simulink model "ES008A_PwrSply"  (R2013b)
settings: Solver=FixedStepDiscrete  SolverMode=SingleTasking  StartTime=0.0  StopTime=1  FixedStep=0.002  RelTol=1e-3
values from neighbouring files (symbols this model uses):
  DiagcReg0Err = DataDict.NTC    [ES008A_PwrSply_DataDict.m]
  DiagcReg1Err = DataDict.NTC    [ES008A_PwrSply_DataDict.m]
  PWRSPLYDIAGREG0READVAL_CNT_U16 = DataDict.Constant    [ES008A_PwrSply_DataDict.m]
  PWRSPLYDIAGREG1READVAL_CNT_U16 = DataDict.Constant    [ES008A_PwrSply_DataDict.m]
  PwrSplyNtc0x07BFailStep = DataDict.Calibration    [ES008A_PwrSply_DataDict.m]
  PwrSplyNtc0x07BPassStep = DataDict.Calibration    [ES008A_PwrSply_DataDict.m]
  PwrSplyNtc0x07CFailStep = DataDict.Calibration    [ES008A_PwrSply_DataDict.m]
  PwrSplyNtc0x07CPassStep = DataDict.Calibration    [ES008A_PwrSply_DataDict.m]
  PwrSplyNtc0x07DFailStep = DataDict.Calibration    [ES008A_PwrSply_DataDict.m]
  PwrSplyNtc0x07DPassStep = DataDict.Calibration    [ES008A_PwrSply_DataDict.m]
  PWRSPLYOUTPENAWRVAL_CNT_U16 = DataDict.Constant    [ES008A_PwrSply_DataDict.m]
  PWRSPLYVRFYRESREG0READVAL_CNT_U16 = DataDict.Constant    [ES008A_PwrSply_DataDict.m]
  PWRSPLYVRFYRESREG1READVAL_CNT_U16 = DataDict.Constant    [ES008A_PwrSply_DataDict.m]
  SerlErr = DataDict.NTC    [ES008A_PwrSply_DataDict.m]
  SpiConf_SpiChannel_PwrSplyCh1 = DataDict.Constant    [ES008A_PwrSply_DataDict.m]
  SpiConf_SpiChannel_PwrSplyCh2 = DataDict.Constant    [ES008A_PwrSply_DataDict.m]
  SpiConf_SpiChannel_PwrSplyCh3 = DataDict.Constant    [ES008A_PwrSply_DataDict.m]
  SpiConf_SpiChannel_PwrSplyCh4 = DataDict.Constant    [ES008A_PwrSply_DataDict.m]
  SpiConf_SpiChannel_PwrSplyCh5 = DataDict.Constant    [ES008A_PwrSply_DataDict.m]
  SpiConf_SpiSequence_PwrSplySeq1 = DataDict.Constant    [ES008A_PwrSply_DataDict.m]
  SpiConf_SpiSequence_PwrSplySeq2 = DataDict.Constant    [ES008A_PwrSply_DataDict.m]
  SpiConf_SpiSequence_PwrSplySeq3 = DataDict.Constant    [ES008A_PwrSply_DataDict.m]
  SpiConf_SpiSequence_PwrSplySeq4 = DataDict.Constant    [ES008A_PwrSply_DataDict.m]
  SpiConf_SpiSequence_PwrSplySeq5 = DataDict.Constant    [ES008A_PwrSply_DataDict.m]
  StrtUpSelfTestReg0Err = DataDict.NTC    [ES008A_PwrSply_DataDict.m]
  StrtUpSelfTestReg1Err = DataDict.NTC    [ES008A_PwrSply_DataDict.m]
undefined symbols (not defined in the file or in its folder): sigbuilder_block, SysSt1
libraries: simulink x11
(part 3 of 4)

== system ES008A_PwrSply/PwrSply/PwrSplyPer1/SysSt = Warm Init OR Enable/PwrSplyReadWrOrderFlg2 = 0 (Write Cmd to get Diag Status) /Read Message 1/Call_Spi_AsyncTransmit ==
  Sequence : Inport
  CopyRight1 : Subsystem  Description=|  mask(Copyright Information){none=on}
      | Copyright info block.                                               
      |                                                                     
      | Place copyright information at the top of every subsystem in design.
      mask prompts: none "No parameters"
      mask help: Place copyright information at the top of every subsystem in design.
      mask Display:
      | NxtrConf = 'Nexteer Confidential';
      | 
      | sys = bdroot; %handle for the current model ("system")
      | first = get_param(sys,'Created');
      | first = first(end-3:end);  %year is last four digits
      | 
      | last = get_param(sys,'LastModifiedDate');
      | if isempty(last)
      |     last = datestr(now,'yyyy');
      | else
      |     last = last(end-3:end);
      | end
      | 
      | if strcmp(first,last)
      |     fprintf('%s -- Copyright %s Nexteer',NxtrConf,first)
      | else
      |     fprintf('%s -- %s%s- %s Nexteer',NxtrConf,char(169),first,last)
      | end
  Terminator : Terminator
  wires:
  Sequence/1 -> Terminator/1

== system ES008A_PwrSply/PwrSply/PwrSplyPer1/SysSt = Warm Init OR Enable/PwrSplyReadWrOrderFlg2 = 0 (Write Cmd to get Diag Status) /Read Message 1/CopyRight1 ==

== system ES008A_PwrSply/PwrSply/PwrSplyPer1/SysSt = Warm Init OR Enable/PwrSplyReadWrOrderFlg2 = 0 (Write Cmd to get Diag Status) /Read Message 1/Spi_WriteIB ==
  Channel : Inport
  DataBufferPtr : Inport  Port=2
  CopyRight1 : Subsystem  Description=|  mask(Copyright Information){none=on}
      | Copyright info block.                                               
      |                                                                     
      | Place copyright information at the top of every subsystem in design.
      mask prompts: none "No parameters"
      mask help: Place copyright information at the top of every subsystem in design.
      mask Display:
      | NxtrConf = 'Nexteer Confidential';
      | 
      | sys = bdroot; %handle for the current model ("system")
      | first = get_param(sys,'Created');
      | first = first(end-3:end);  %year is last four digits
      | 
      | last = get_param(sys,'LastModifiedDate');
      | if isempty(last)
      |     last = datestr(now,'yyyy');
      | else
      |     last = last(end-3:end);
      | end
      | 
      | if strcmp(first,last)
      |     fprintf('%s -- Copyright %s Nexteer',NxtrConf,first)
      | else
      |     fprintf('%s -- %s%s- %s Nexteer',NxtrConf,char(169),first,last)
      | end
  Terminator : Terminator
  Terminator1 : Terminator
  wires:
  DataBufferPtr/1 -> Terminator1/1
  Channel/1 -> Terminator/1

== system ES008A_PwrSply/PwrSply/PwrSplyPer1/SysSt = Warm Init OR Enable/PwrSplyReadWrOrderFlg2 = 0 (Write Cmd to get Diag Status) /Read Message 2/Call_Spi_AsyncTransmit ==
  Sequence : Inport
  CopyRight1 : Subsystem  Description=|  mask(Copyright Information){none=on}
      | Copyright info block.                                               
      |                                                                     
      | Place copyright information at the top of every subsystem in design.
      mask prompts: none "No parameters"
      mask help: Place copyright information at the top of every subsystem in design.
      mask Display:
      | NxtrConf = 'Nexteer Confidential';
      | 
      | sys = bdroot; %handle for the current model ("system")
      | first = get_param(sys,'Created');
      | first = first(end-3:end);  %year is last four digits
      | 
      | last = get_param(sys,'LastModifiedDate');
      | if isempty(last)
      |     last = datestr(now,'yyyy');
      | else
      |     last = last(end-3:end);
      | end
      | 
      | if strcmp(first,last)
      |     fprintf('%s -- Copyright %s Nexteer',NxtrConf,first)
      | else
      |     fprintf('%s -- %s%s- %s Nexteer',NxtrConf,char(169),first,last)
      | end
  Terminator : Terminator
  wires:
  Sequence/1 -> Terminator/1

== system ES008A_PwrSply/PwrSply/PwrSplyPer1/SysSt = Warm Init OR Enable/PwrSplyReadWrOrderFlg2 = 0 (Write Cmd to get Diag Status) /Read Message 2/CopyRight1 ==

== system ES008A_PwrSply/PwrSply/PwrSplyPer1/SysSt = Warm Init OR Enable/PwrSplyReadWrOrderFlg2 = 0 (Write Cmd to get Diag Status) /Read Message 2/Spi_WriteIB ==
  Channel : Inport
  DataBufferPtr : Inport  Port=2
  CopyRight1 : Subsystem  Description=|  mask(Copyright Information){none=on}
      | Copyright info block.                                               
      |                                                                     
      | Place copyright information at the top of every subsystem in design.
      mask prompts: none "No parameters"
      mask help: Place copyright information at the top of every subsystem in design.
      mask Display:
      | NxtrConf = 'Nexteer Confidential';
      | 
      | sys = bdroot; %handle for the current model ("system")
      | first = get_param(sys,'Created');
      | first = first(end-3:end);  %year is last four digits
      | 
      | last = get_param(sys,'LastModifiedDate');
      | if isempty(last)
      |     last = datestr(now,'yyyy');
      | else
      |     last = last(end-3:end);
      | end
      | 
      | if strcmp(first,last)
      |     fprintf('%s -- Copyright %s Nexteer',NxtrConf,first)
      | else
      |     fprintf('%s -- %s%s- %s Nexteer',NxtrConf,char(169),first,last)
      | end
  Terminator : Terminator
  Terminator1 : Terminator
  wires:
  Channel/1 -> Terminator/1
  DataBufferPtr/1 -> Terminator1/1

== system ES008A_PwrSply/PwrSply/PwrSplyPer1/SysSt = Warm Init OR Enable/PwrSplyReadWrOrderFlg2 = 1 (Read Buffer)/Channel 4/CH 4 // Verify Result Reg 0 - NTCNR_0X07E (V5A, V5CAN, 3V3, BUCK) ==
  note: Channel 4 --> for Verify_Result_0 Register
      | Channel 5 --> for Verify_Result_1 Register
  NtcStsInfo : Inport
  Action Port : ActionPort  ActionType=then
  Bitwise Operator1 : simulink/Logic and Bit Operations/Bitwise Operator  logicop=NOT  UseBitMask=off  BitMask=bin2dec('11011001')  BitMaskRealWorld=Stored Integer
  CopyRight1 : Subsystem  Description=|  mask(Copyright Information){none=on}
      | Copyright info block.                                               
      |                                                                     
      | Place copyright information at the top of every subsystem in design.
      mask prompts: none "No parameters"
      mask help: Place copyright information at the top of every subsystem in design.
      mask Display:
      | NxtrConf = 'Nexteer Confidential';
      | 
      | sys = bdroot; %handle for the current model ("system")
      | first = get_param(sys,'Created');
      | first = first(end-3:end);  %year is last four digits
      | 
      | last = get_param(sys,'LastModifiedDate');
      | if isempty(last)
      |     last = datestr(now,'yyyy');
      | else
      |     last = last(end-3:end);
      | end
      | 
      | if strcmp(first,last)
      |     fprintf('%s -- Copyright %s Nexteer',NxtrConf,first)
      | else
      |     fprintf('%s -- %s%s- %s Nexteer',NxtrConf,char(169),first,last)
      | end
  Ground : Ground
  NtcNr : Constant  Value=StrtUpSelfTestReg0Err
  NtcSts : Constant  OutDataTypeStr=uint8
  SetNtcSts : Subsystem  RequirementInfo={'linktype_rmi_doors' '0000cf50 (/ESG Group/FDD Module Requirements/EA4 Specific/ES008A_PwrSply)' '#ES008A_128' 'true' 'REQ: ES008A_128' '' ; 'linktype_rmi_doors' '0000cf50 (/ESG Group/FDD Module Requirements/EA4 Specific/ES008A_PwrSply)' '#ES008A_129' 'true' 'REQ: ES008A_129' '' ; 'linktype_rmi_doors' '0000cf50 (/ESG Group/FDD Module Requirements/EA4 Specific/ES008A_PwrSply)' '#ES008A_135' 'true' 'REQ: ES008A_135' '' ; 'linktype_rmi_doors' '0000cf50 (/ESG Group/FDD Module Requirements/EA4 Specific/ES008A_PwrSply)' '#ES008A_134' 'true' 'REQ: ES008A_134' '' ; 'linktype_rmi_doors' '0000cf50 (/ESG Group/FDD Module Requirements/EA4 Specific/ES008A_PwrSply)' '#ES008A_133' 'true' 'REQ: ES008A_133' '' ; 'linktype_rmi_doors' '0000cf50 (/ESG Group/FDD Module Requirements/EA4 Specific/ES008A_PwrSply)' '#ES008A_132' 'true' 'REQ: ES008A_132' '' ; 'linktype_rmi_doors' '0000cf50 (/ESG Group/FDD Module Requirements/EA4 Specific/ES008A_PwrSply)' '#ES008A_131' 'true' 'REQ: ES008A_131' '' ; 'linktype_rmi_doors' '0000cf50 (/ESG Group/FDD Module Requirements/EA4 Specific/ES008A_PwrSply)' '#ES008A_130' 'true' 'REQ: ES008A_130' '' } %GIDa_275bfab4_ec12_4082_a419_c11eb7b6dec0
  wires:
  NtcStsInfo/1 -> Bitwise Operator1/1
  Ground/1 -> SetNtcSts/4(DebStep)
  NtcSts/1 -> SetNtcSts/3(NtcSts)
  Bitwise Operator1/1 -> SetNtcSts/2(NtcStInfo)
  NtcNr/1 -> SetNtcSts/1(NtcNr)

== system ES008A_PwrSply/PwrSply/PwrSplyPer1/SysSt = Warm Init OR Enable/PwrSplyReadWrOrderFlg2 = 1 (Read Buffer)/Channel 4/CopyRight1 ==

== system ES008A_PwrSply/PwrSply/PwrSplyPer1/SysSt = Warm Init OR Enable/PwrSplyReadWrOrderFlg2 = 1 (Read Buffer)/Channel 4/No Startup Test Error 0 ==
  Action Port : ActionPort  ActionType=else
  CopyRight1 : Subsystem  Description=|  mask(Copyright Information){none=on}
      | Copyright info block.                                               
      |                                                                     
      | Place copyright information at the top of every subsystem in design.
      mask prompts: none "No parameters"
      mask help: Place copyright information at the top of every subsystem in design.
      mask Display:
      | NxtrConf = 'Nexteer Confidential';
      | 
      | sys = bdroot; %handle for the current model ("system")
      | first = get_param(sys,'Created');
      | first = first(end-3:end);  %year is last four digits
      | 
      | last = get_param(sys,'LastModifiedDate');
      | if isempty(last)
      |     last = datestr(now,'yyyy');
      | else
      |     last = last(end-3:end);
      | end
      | 
      | if strcmp(first,last)
      |     fprintf('%s -- Copyright %s Nexteer',NxtrConf,first)
      | else
      |     fprintf('%s -- %s%s- %s Nexteer',NxtrConf,char(169),first,last)
      | end
  Ground : Ground
  NtcNr : Constant  Value=StrtUpSelfTestReg0Err
  NtcSts : Constant  Value=0  OutDataTypeStr=uint8
  NtcStsInfo : Constant  Value=0  OutDataTypeStr=uint8
  SetNtcSts : Subsystem  RequirementInfo={'linktype_rmi_doors' '0000cf50 (/ESG Group/FDD Module Requirements/EA4 Specific/ES008A_PwrSply)' '#ES008A_124' 'true' 'REQ: ES008A_124' '' } %GIDa_e0576653_0d47_4805_9c34_52b8011502e8
  wires:
  NtcStsInfo/1 -> SetNtcSts/2(NtcStInfo)
  NtcNr/1 -> SetNtcSts/1(NtcNr)
  Ground/1 -> SetNtcSts/4(DebStep)
  NtcSts/1 -> SetNtcSts/3(NtcSts)

== system ES008A_PwrSply/PwrSply/PwrSplyPer1/SysSt = Warm Init OR Enable/PwrSplyReadWrOrderFlg2 = 1 (Read Buffer)/Channel 4/Spi_ReadIB ==
  note: Read Buffer - Simulation Purpose Only
      |
      |
      |
      |               XXXX XXXX 1111 1111
  note: 001011111111110
  Channel : Inport
  Constant3 : Constant  Value=255  OutDataTypeStr=uint16
  CopyRight1 : Subsystem  Description=|  mask(Copyright Information){none=on}
      | Copyright info block.                                               
      |                                                                     
      | Place copyright information at the top of every subsystem in design.
      mask prompts: none "No parameters"
      mask help: Place copyright information at the top of every subsystem in design.
      mask Display:
      | NxtrConf = 'Nexteer Confidential';
      | 
      | sys = bdroot; %handle for the current model ("system")
      | first = get_param(sys,'Created');
      | first = first(end-3:end);  %year is last four digits
      | 
      | last = get_param(sys,'LastModifiedDate');
      | if isempty(last)
      |     last = datestr(now,'yyyy');
      | else
      |     last = last(end-3:end);
      | end
      | 
      | if strcmp(first,last)
      |     fprintf('%s -- Copyright %s Nexteer',NxtrConf,first)
      | else
      |     fprintf('%s -- %s%s- %s Nexteer',NxtrConf,char(169),first,last)
      | end
  Terminator : Terminator
  Rx : Outport
  wires:
  Channel/1 -> Terminator/1
  Constant3/1 -> Rx/1

== system ES008A_PwrSply/PwrSply/PwrSplyPer1/SysSt = Warm Init OR Enable/PwrSplyReadWrOrderFlg2 = 1 (Read Buffer)/Channel 5/CH 5 // Verify Result Reg 1 - NTCNR_0X07F (VREG, V5P, V5B) ==
  note: Channel 4 --> for Verify_Result_0 Register
      | Channel 5 --> for Verify_Result_1 Register
  NtcStsInfo : Inport
  Action Port : ActionPort  ActionType=then
  Bitwise Operator1 : simulink/Logic and Bit Operations/Bitwise Operator  logicop=NOT  UseBitMask=off  BitMask=bin2dec('11011001')  BitMaskRealWorld=Stored Integer
  CopyRight1 : Subsystem  Description=|  mask(Copyright Information){none=on}
      | Copyright info block.                                               
      |                                                                     
      | Place copyright information at the top of every subsystem in design.
      mask prompts: none "No parameters"
      mask help: Place copyright information at the top of every subsystem in design.
      mask Display:
      | NxtrConf = 'Nexteer Confidential';
      | 
      | sys = bdroot; %handle for the current model ("system")
      | first = get_param(sys,'Created');
      | first = first(end-3:end);  %year is last four digits
      | 
      | last = get_param(sys,'LastModifiedDate');
      | if isempty(last)
      |     last = datestr(now,'yyyy');
      | else
      |     last = last(end-3:end);
      | end
      | 
      | if strcmp(first,last)
      |     fprintf('%s -- Copyright %s Nexteer',NxtrConf,first)
      | else
      |     fprintf('%s -- %s%s- %s Nexteer',NxtrConf,char(169),first,last)
      | end
  Ground : Ground
  NtcNr : Constant  Value=StrtUpSelfTestReg1Err
  NtcSts : Constant  OutDataTypeStr=uint8
  SetNtcSts : Subsystem  RequirementInfo={'linktype_rmi_doors' '0000cf50 (/ESG Group/FDD Module Requirements/EA4 Specific/ES008A_PwrSply)' '#ES008A_136' 'true' 'REQ: ES008A_136' '' ; 'linktype_rmi_doors' '0000cf50 (/ESG Group/FDD Module Requirements/EA4 Specific/ES008A_PwrSply)' '#ES008A_137' 'true' 'REQ: ES008A_137' '' ; 'linktype_rmi_doors' '0000cf50 (/ESG Group/FDD Module Requirements/EA4 Specific/ES008A_PwrSply)' '#ES008A_141' 'true' 'REQ: ES008A_141' '' ; 'linktype_rmi_doors' '0000cf50 (/ESG Group/FDD Module Requirements/EA4 Specific/ES008A_PwrSply)' '#ES008A_140' 'true' 'REQ: ES008A_140' '' ; 'linktype_rmi_doors' '0000cf50 (/ESG Group/FDD Module Requirements/EA4 Specific/ES008A_PwrSply)' '#ES008A_139' 'true' 'REQ: ES008A_139' '' ; 'linktype_rmi_doors' '0000cf50 (/ESG Group/FDD Module Requirements/EA4 Specific/ES008A_PwrSply)' '#ES008A_138' 'true' 'REQ: ES008A_138' '' ; 'linktype_rmi_doors' '0000cf50 (/ESG Group/FDD Module Requirements/EA4 Specific/ES008A_PwrSply)' '#ES008A_49' 'true' 'REQ: ES008A_49' '' ; 'linktype_rmi_doors' '0000cf50 (/ESG Group/FDD Module Requirements/EA4 Specific/ES008A_PwrSply)' '#ES008A_49' 'true' 'REQ: ES008A_49' '' } %GIDa_cbc9c02c_b5d9_4897_b1c2_1afec5aef5e7
  wires:
  NtcStsInfo/1 -> Bitwise Operator1/1
  NtcNr/1 -> SetNtcSts/1(NtcNr)
  Ground/1 -> SetNtcSts/4(DebStep)
  NtcSts/1 -> SetNtcSts/3(NtcSts)
  Bitwise Operator1/1 -> SetNtcSts/2(NtcStInfo)

== system ES008A_PwrSply/PwrSply/PwrSplyPer1/SysSt = Warm Init OR Enable/PwrSplyReadWrOrderFlg2 = 1 (Read Buffer)/Channel 5/CopyRight1 ==

== system ES008A_PwrSply/PwrSply/PwrSplyPer1/SysSt = Warm Init OR Enable/PwrSplyReadWrOrderFlg2 = 1 (Read Buffer)/Channel 5/No Startup Test Error 1 ==
  Action Port : ActionPort  ActionType=else
  CopyRight1 : Subsystem  Description=|  mask(Copyright Information){none=on}
      | Copyright info block.                                               
      |                                                                     
      | Place copyright information at the top of every subsystem in design.
      mask prompts: none "No parameters"
      mask help: Place copyright information at the top of every subsystem in design.
      mask Display:
      | NxtrConf = 'Nexteer Confidential';
      | 
      | sys = bdroot; %handle for the current model ("system")
      | first = get_param(sys,'Created');
      | first = first(end-3:end);  %year is last four digits
      | 
      | last = get_param(sys,'LastModifiedDate');
      | if isempty(last)
      |     last = datestr(now,'yyyy');
      | else
      |     last = last(end-3:end);
      | end
      | 
      | if strcmp(first,last)
      |     fprintf('%s -- Copyright %s Nexteer',NxtrConf,first)
      | else
      |     fprintf('%s -- %s%s- %s Nexteer',NxtrConf,char(169),first,last)
      | end
  Ground : Ground
  NtcNr : Constant  Value=StrtUpSelfTestReg1Err
  NtcSts : Constant  Value=0  OutDataTypeStr=uint8
  NtcStsInfo : Constant  Value=0  OutDataTypeStr=uint8
  SetNtcSts : Subsystem  RequirementInfo={'linktype_rmi_doors' '0000cf50 (/ESG Group/FDD Module Requirements/EA4 Specific/ES008A_PwrSply)' '#ES008A_125' 'true' 'REQ: ES008A_125' '' } %GIDa_9009c51d_1145_40b1_96ca_5dc7a0ec55a9
  wires:
  NtcStsInfo/1 -> SetNtcSts/2(NtcStInfo)
  NtcNr/1 -> SetNtcSts/1(NtcNr)
  Ground/1 -> SetNtcSts/4(DebStep)
  NtcSts/1 -> SetNtcSts/3(NtcSts)

== system ES008A_PwrSply/PwrSply/PwrSplyPer1/SysSt = Warm Init OR Enable/PwrSplyReadWrOrderFlg2 = 1 (Read Buffer)/Channel 5/Spi_ReadIB ==
  note: 001011111111110
  note: Read Buffer - Simulation Purpose Only
  Channel : Inport
  Constant3 : Constant  Value=44  OutDataTypeStr=uint16
  CopyRight1 : Subsystem  Description=|  mask(Copyright Information){none=on}
      | Copyright info block.                                               
      |                                                                     
      | Place copyright information at the top of every subsystem in design.
      mask prompts: none "No parameters"
      mask help: Place copyright information at the top of every subsystem in design.
      mask Display:
      | NxtrConf = 'Nexteer Confidential';
      | 
      | sys = bdroot; %handle for the current model ("system")
      | first = get_param(sys,'Created');
      | first = first(end-3:end);  %year is last four digits
      | 
      | last = get_param(sys,'LastModifiedDate');
      | if isempty(last)
      |     last = datestr(now,'yyyy');
      | else
      |     last = last(end-3:end);
      | end
      | 
      | if strcmp(first,last)
      |     fprintf('%s -- Copyright %s Nexteer',NxtrConf,first)
      | else
      |     fprintf('%s -- %s%s- %s Nexteer',NxtrConf,char(169),first,last)
      | end
  Terminator : Terminator
  Rx : Outport
  wires:
  Constant3/1 -> Rx/1
  Channel/1 -> Terminator/1

== system ES008A_PwrSply/PwrSply/PwrSplyPer1/SysSt = Enable/PwrSplyReadWrOrderFlg1 = 0 (Write Cmd to get Diag Status) /Read Message 1/Call_Spi_AsyncTransmit/CopyRight1 ==

== system ES008A_PwrSply/PwrSply/PwrSplyPer1/SysSt = Enable/PwrSplyReadWrOrderFlg1 = 0 (Write Cmd to get Diag Status) /Read Message 1/Spi_WriteIB/CopyRight1 ==

== system ES008A_PwrSply/PwrSply/PwrSplyPer1/SysSt = Enable/PwrSplyReadWrOrderFlg1 = 0 (Write Cmd to get Diag Status) /Read Message 2/Call_Spi_AsyncTransmit/CopyRight1 ==

== system ES008A_PwrSply/PwrSply/PwrSplyPer1/SysSt = Enable/PwrSplyReadWrOrderFlg1 = 0 (Write Cmd to get Diag Status) /Read Message 2/Spi_WriteIB/CopyRight1 ==

== system ES008A_PwrSply/PwrSply/PwrSplyPer1/SysSt = Enable/PwrSplyReadWrOrderFlg1 = 0 (Write Cmd to get Diag Status) /Write Message 1/Call_Spi_AsyncTransmit/CopyRight1 ==

== system ES008A_PwrSply/PwrSply/PwrSplyPer1/SysSt = Enable/PwrSplyReadWrOrderFlg1 = 0 (Write Cmd to get Diag Status) /Write Message 1/Spi_WriteIB/CopyRight1 ==

== system ES008A_PwrSply/PwrSply/PwrSplyPer1/SysSt = Enable/PwrSplyReadWrOrderFlg1 = 1 (Read Buffer)/CH 2 // Diag Reg 0 Error - NTCNR_0X07C (V5P, V5A, V5B, V5CAN)/SetNtcSts/CopyRight2 ==

== system ES008A_PwrSply/PwrSply/PwrSplyPer1/SysSt = Enable/PwrSplyReadWrOrderFlg1 = 1 (Read Buffer)/CH 2 // Diag Reg 0 Error - NTCNR_0X07C (V5P, V5A, V5B, V5CAN)/Spi_ReadIB/CopyRight1 ==

== system ES008A_PwrSply/PwrSply/PwrSplyPer1/SysSt = Enable/PwrSplyReadWrOrderFlg1 = 1 (Read Buffer)/CH 3 // Diag Reg 1 Error - NTCNR_0X07B (VREG, BUCK, V3V3)/SetNtcSts/CopyRight2 ==

== system ES008A_PwrSply/PwrSply/PwrSplyPer1/SysSt = Enable/PwrSplyReadWrOrderFlg1 = 1 (Read Buffer)/CH 3 // Diag Reg 1 Error - NTCNR_0X07B (VREG, BUCK, V3V3)/Spi_ReadIB/CopyRight1 ==

== system ES008A_PwrSply/PwrSply/PwrSplyPer1/SysSt = Enable/PwrSplyReadWrOrderFlg1 = 1 (Read Buffer)/No  Error - Diag Reg 0/SetNtcSts/CopyRight2 ==

== system ES008A_PwrSply/PwrSply/PwrSplyPer1/SysSt = Enable/PwrSplyReadWrOrderFlg1 = 1 (Read Buffer)/No  Error - Diag Reg 1/SetNtcSts/CopyRight2 ==

== system ES008A_PwrSply/PwrSply/PwrSplyPer1/SysSt = Enable/PwrSplyReadWrOrderFlg1 = 1 (Read Buffer)/No Serial Error/SetNtcSts/CopyRight2 ==

== system ES008A_PwrSply/PwrSply/PwrSplyPer1/SysSt = Enable/PwrSplyReadWrOrderFlg1 = 1 (Read Buffer)/Serial Error - NTCNR_0X07D/SetNtcSts/CopyRight2 ==

== system ES008A_PwrSply/PwrSply/PwrSplyPer1/SysSt = Warm Init OR Enable/PwrSplyReadWrOrderFlg2 = 0 (Write Cmd to get Diag Status) /Read Message 1/Call_Spi_AsyncTransmit/CopyRight1 ==

== system ES008A_PwrSply/PwrSply/PwrSplyPer1/SysSt = Warm Init OR Enable/PwrSplyReadWrOrderFlg2 = 0 (Write Cmd to get Diag Status) /Read Message 1/Spi_WriteIB/CopyRight1 ==

== system ES008A_PwrSply/PwrSply/PwrSplyPer1/SysSt = Warm Init OR Enable/PwrSplyReadWrOrderFlg2 = 0 (Write Cmd to get Diag Status) /Read Message 2/Call_Spi_AsyncTransmit/CopyRight1 ==

== system ES008A_PwrSply/PwrSply/PwrSplyPer1/SysSt = Warm Init OR Enable/PwrSplyReadWrOrderFlg2 = 0 (Write Cmd to get Diag Status) /Read Message 2/Spi_WriteIB/CopyRight1 ==

== system ES008A_PwrSply/PwrSply/PwrSplyPer1/SysSt = Warm Init OR Enable/PwrSplyReadWrOrderFlg2 = 1 (Read Buffer)/Channel 4/CH 4 // Verify Result Reg 0 - NTCNR_0X07E (V5A, V5CAN, 3V3, BUCK)/CopyRight1 ==

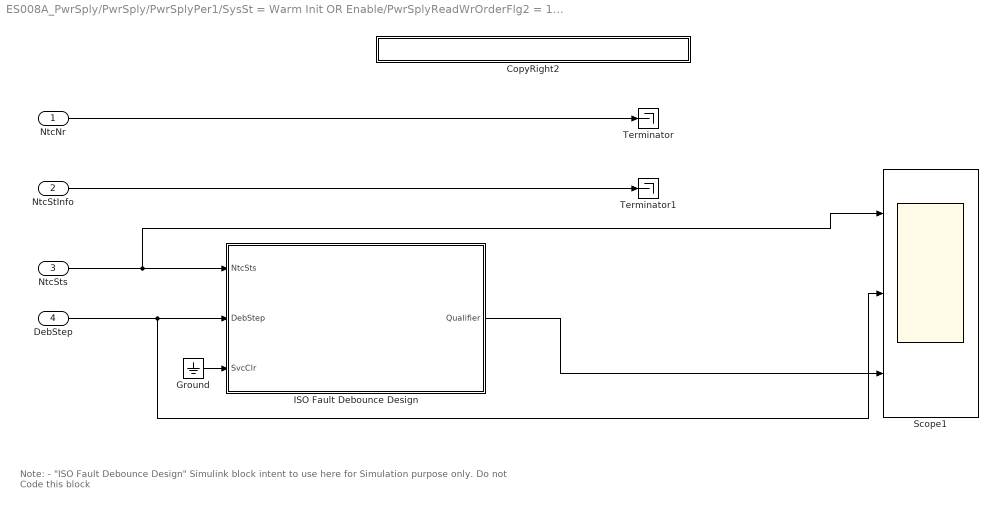
== system ES008A_PwrSply/PwrSply/PwrSplyPer1/SysSt = Warm Init OR Enable/PwrSplyReadWrOrderFlg2 = 1 (Read Buffer)/Channel 4/CH 4 // Verify Result Reg 0 - NTCNR_0X07E (V5A, V5CAN, 3V3, BUCK)/SetNtcSts ==
  note: Note:
      |
      | - "ISO Fault Debounce Design" Simulink block intent to use here for Simulation purpose only. Do not Code this block
  NtcNr : Inport
  NtcStInfo : Inport  Port=2
  NtcSts : Inport  Port=3  OutDataTypeStr=uint8
  DebStep : Inport  Port=4  OutDataTypeStr=uint16
  CopyRight2 : Subsystem  Description=|  mask(Copyright Information){none=on}
      | Copyright info block.                                               
      |                                                                     
      | Place copyright information at the top of every subsystem in design.
      mask prompts: none "No parameters"
      mask help: Place copyright information at the top of every subsystem in design.
      mask Display:
      | NxtrConf = 'Nexteer Confidential';
      | 
      | sys = bdroot; %handle for the current model ("system")
      | first = get_param(sys,'Created');
      | first = first(end-3:end);  %year is last four digits
      | 
      | last = get_param(sys,'LastModifiedDate');
      | if isempty(last)
      |     last = datestr(now,'yyyy');
      | else
      |     last = last(end-3:end);
      | end
      | 
      | if strcmp(first,last)
      |     fprintf('%s -- Copyright %s Nexteer',NxtrConf,first)
      | else
      |     fprintf('%s -- %s%s- %s Nexteer',NxtrConf,char(169),first,last)
      | end
  Ground : Ground
  ISO Fault Debounce Design : Stateflow chart  TreatAsAtomicUnit=on
      settings: AttributesFormatString=|
      | Simulation Purpose Only.
      | Do Not Code this block
      | Diagnostic Manager Owns this requirement
  Scope1 : Scope  NumInputPorts=3
      settings: YMin=-5~-5~-5  YMax=5~5~5  SaveName=ScopeData5
  Terminator : Terminator
  Terminator1 : Terminator
  wires:
  NtcStInfo/1 -> Terminator1/1
  NtcNr/1 -> Terminator/1
  NtcSts/1 -> ISO Fault Debounce Design/1(NtcSts), Scope1/1
  DebStep/1 -> ISO Fault Debounce Design/2(DebStep), Scope1/2
  ISO Fault Debounce Design/1(Qualifier) -> Scope1/3
  Ground/1 -> ISO Fault Debounce Design/3(SvcClr)

== system ES008A_PwrSply/PwrSply/PwrSplyPer1/SysSt = Warm Init OR Enable/PwrSplyReadWrOrderFlg2 = 1 (Read Buffer)/Channel 4/No Startup Test Error 0/CopyRight1 ==

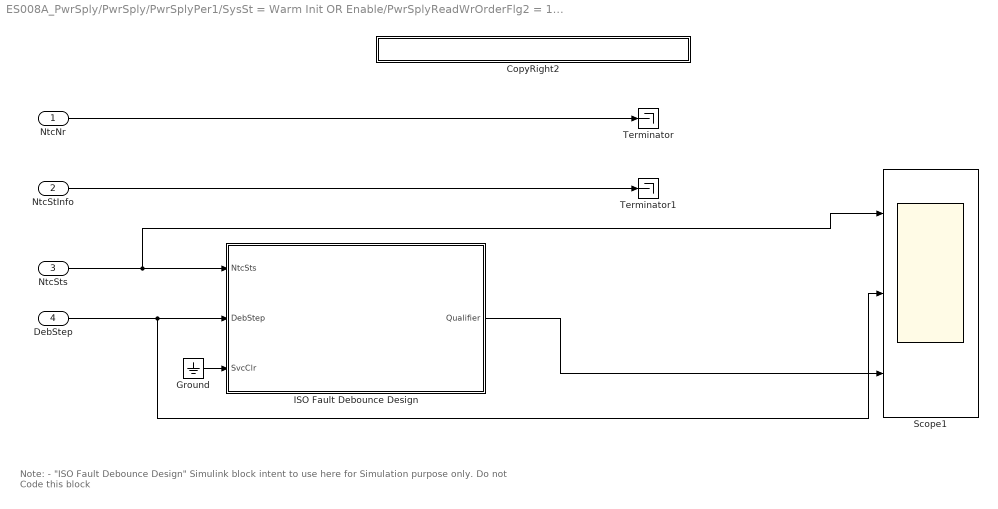
== system ES008A_PwrSply/PwrSply/PwrSplyPer1/SysSt = Warm Init OR Enable/PwrSplyReadWrOrderFlg2 = 1 (Read Buffer)/Channel 4/No Startup Test Error 0/SetNtcSts ==
  note: Note:
      |
      | - "ISO Fault Debounce Design" Simulink block intent to use here for Simulation purpose only. Do not Code this block
  NtcNr : Inport
  NtcStInfo : Inport  Port=2
  NtcSts : Inport  Port=3  OutDataTypeStr=uint8
  DebStep : Inport  Port=4  OutDataTypeStr=uint16
  CopyRight2 : Subsystem  Description=|  mask(Copyright Information){none=on}
      | Copyright info block.                                               
      |                                                                     
      | Place copyright information at the top of every subsystem in design.
      mask prompts: none "No parameters"
      mask help: Place copyright information at the top of every subsystem in design.
      mask Display:
      | NxtrConf = 'Nexteer Confidential';
      | 
      | sys = bdroot; %handle for the current model ("system")
      | first = get_param(sys,'Created');
      | first = first(end-3:end);  %year is last four digits
      | 
      | last = get_param(sys,'LastModifiedDate');
      | if isempty(last)
      |     last = datestr(now,'yyyy');
      | else
      |     last = last(end-3:end);
      | end
      | 
      | if strcmp(first,last)
      |     fprintf('%s -- Copyright %s Nexteer',NxtrConf,first)
      | else
      |     fprintf('%s -- %s%s- %s Nexteer',NxtrConf,char(169),first,last)
      | end
  Ground : Ground
  ISO Fault Debounce Design : Stateflow chart  TreatAsAtomicUnit=on
      settings: AttributesFormatString=|
      | Simulation Purpose Only.
      | Do Not Code this block
      | Diagnostic Manager Owns this requirement
  Scope1 : Scope  NumInputPorts=3
      settings: YMin=-5~-5~-5  YMax=5~5~5  SaveName=ScopeData5
  Terminator : Terminator
  Terminator1 : Terminator
  wires:
  NtcStInfo/1 -> Terminator1/1
  NtcNr/1 -> Terminator/1
  NtcSts/1 -> ISO Fault Debounce Design/1(NtcSts), Scope1/1
  DebStep/1 -> ISO Fault Debounce Design/2(DebStep), Scope1/2
  ISO Fault Debounce Design/1(Qualifier) -> Scope1/3
  Ground/1 -> ISO Fault Debounce Design/3(SvcClr)

== system ES008A_PwrSply/PwrSply/PwrSplyPer1/SysSt = Warm Init OR Enable/PwrSplyReadWrOrderFlg2 = 1 (Read Buffer)/Channel 4/Spi_ReadIB/CopyRight1 ==

== system ES008A_PwrSply/PwrSply/PwrSplyPer1/SysSt = Warm Init OR Enable/PwrSplyReadWrOrderFlg2 = 1 (Read Buffer)/Channel 5/CH 5 // Verify Result Reg 1 - NTCNR_0X07F (VREG, V5P, V5B)/CopyRight1 ==

== system ES008A_PwrSply/PwrSply/PwrSplyPer1/SysSt = Warm Init OR Enable/PwrSplyReadWrOrderFlg2 = 1 (Read Buffer)/Channel 5/CH 5 // Verify Result Reg 1 - NTCNR_0X07F (VREG, V5P, V5B)/SetNtcSts ==
  note: Note:
      |
      | - "ISO Fault Debounce Design" Simulink block intent to use here for Simulation purpose only. Do not Code this block
  NtcNr : Inport
  NtcStInfo : Inport  Port=2
  NtcSts : Inport  Port=3  OutDataTypeStr=uint8
  DebStep : Inport  Port=4  OutDataTypeStr=uint16
  CopyRight2 : Subsystem  Description=|  mask(Copyright Information){none=on}
      | Copyright info block.                                               
      |                                                                     
      | Place copyright information at the top of every subsystem in design.
      mask prompts: none "No parameters"
      mask help: Place copyright information at the top of every subsystem in design.
      mask Display:
      | NxtrConf = 'Nexteer Confidential';
      | 
      | sys = bdroot; %handle for the current model ("system")
      | first = get_param(sys,'Created');
      | first = first(end-3:end);  %year is last four digits
      | 
      | last = get_param(sys,'LastModifiedDate');
      | if isempty(last)
      |     last = datestr(now,'yyyy');
      | else
      |     last = last(end-3:end);
      | end
      | 
      | if strcmp(first,last)
      |     fprintf('%s -- Copyright %s Nexteer',NxtrConf,first)
      | else
      |     fprintf('%s -- %s%s- %s Nexteer',NxtrConf,char(169),first,last)
      | end
  Ground : Ground
  ISO Fault Debounce Design : Stateflow chart  TreatAsAtomicUnit=on
      settings: AttributesFormatString=|
      | Simulation Purpose Only.
      | Do Not Code this block
      | Diagnostic Manager Owns this requirement
  Scope1 : Scope  NumInputPorts=3
      settings: YMin=-5~-5~-5  YMax=5~5~5  SaveName=ScopeData5
  Terminator : Terminator
  Terminator1 : Terminator
  wires:
  NtcStInfo/1 -> Terminator1/1
  NtcNr/1 -> Terminator/1
  NtcSts/1 -> ISO Fault Debounce Design/1(NtcSts), Scope1/1
  DebStep/1 -> ISO Fault Debounce Design/2(DebStep), Scope1/2
  ISO Fault Debounce Design/1(Qualifier) -> Scope1/3
  Ground/1 -> ISO Fault Debounce Design/3(SvcClr)

== system ES008A_PwrSply/PwrSply/PwrSplyPer1/SysSt = Warm Init OR Enable/PwrSplyReadWrOrderFlg2 = 1 (Read Buffer)/Channel 5/No Startup Test Error 1/CopyRight1 ==

== system ES008A_PwrSply/PwrSply/PwrSplyPer1/SysSt = Warm Init OR Enable/PwrSplyReadWrOrderFlg2 = 1 (Read Buffer)/Channel 5/No Startup Test Error 1/SetNtcSts ==
  note: Note:
      |
      | - "ISO Fault Debounce Design" Simulink block intent to use here for Simulation purpose only. Do not Code this block
  NtcNr : Inport
  NtcStInfo : Inport  Port=2
  NtcSts : Inport  Port=3  OutDataTypeStr=uint8
  DebStep : Inport  Port=4  OutDataTypeStr=uint16
  CopyRight2 : Subsystem  Description=|  mask(Copyright Information){none=on}
      | Copyright info block.                                               
      |                                                                     
      | Place copyright information at the top of every subsystem in design.
      mask prompts: none "No parameters"
      mask help: Place copyright information at the top of every subsystem in design.
      mask Display:
      | NxtrConf = 'Nexteer Confidential';
      | 
      | sys = bdroot; %handle for the current model ("system")
      | first = get_param(sys,'Created');
      | first = first(end-3:end);  %year is last four digits
      | 
      | last = get_param(sys,'LastModifiedDate');
      | if isempty(last)
      |     last = datestr(now,'yyyy');
      | else
      |     last = last(end-3:end);
      | end
      | 
      | if strcmp(first,last)
      |     fprintf('%s -- Copyright %s Nexteer',NxtrConf,first)
      | else
      |     fprintf('%s -- %s%s- %s Nexteer',NxtrConf,char(169),first,last)
      | end
  Ground : Ground
  ISO Fault Debounce Design : Stateflow chart  TreatAsAtomicUnit=on
      settings: AttributesFormatString=|
      | Simulation Purpose Only.
      | Do Not Code this block
      | Diagnostic Manager Owns this requirement
  Scope1 : Scope  NumInputPorts=3
      settings: YMin=-5~-5~-5  YMax=5~5~5  SaveName=ScopeData5
  Terminator : Terminator
  Terminator1 : Terminator
  wires:
  NtcStInfo/1 -> Terminator1/1
  NtcNr/1 -> Terminator/1
  NtcSts/1 -> ISO Fault Debounce Design/1(NtcSts), Scope1/1
  DebStep/1 -> ISO Fault Debounce Design/2(DebStep), Scope1/2
  ISO Fault Debounce Design/1(Qualifier) -> Scope1/3
  Ground/1 -> ISO Fault Debounce Design/3(SvcClr)

== system ES008A_PwrSply/PwrSply/PwrSplyPer1/SysSt = Warm Init OR Enable/PwrSplyReadWrOrderFlg2 = 1 (Read Buffer)/Channel 5/Spi_ReadIB/CopyRight1 ==

== system ES008A_PwrSply/PwrSply/PwrSplyPer1/SysSt = Warm Init OR Enable/PwrSplyReadWrOrderFlg2 = 1 (Read Buffer)/Channel 4/CH 4 // Verify Result Reg 0 - NTCNR_0X07E (V5A, V5CAN, 3V3, BUCK)/SetNtcSts/CopyRight2 ==

== system ES008A_PwrSply/PwrSply/PwrSplyPer1/SysSt = Warm Init OR Enable/PwrSplyReadWrOrderFlg2 = 1 (Read Buffer)/Channel 4/No Startup Test Error 0/SetNtcSts/CopyRight2 ==

== system ES008A_PwrSply/PwrSply/PwrSplyPer1/SysSt = Warm Init OR Enable/PwrSplyReadWrOrderFlg2 = 1 (Read Buffer)/Channel 5/CH 5 // Verify Result Reg 1 - NTCNR_0X07F (VREG, V5P, V5B)/SetNtcSts/CopyRight2 ==

== system ES008A_PwrSply/PwrSply/PwrSplyPer1/SysSt = Warm Init OR Enable/PwrSplyReadWrOrderFlg2 = 1 (Read Buffer)/Channel 5/No Startup Test Error 1/SetNtcSts/CopyRight2 ==

== stateflow chart ES008A_PwrSply/PwrSply/PwrSplyPer1/SysSt = Warm Init OR Enable/PwrSplyReadWrOrderFlg2 = 1 (Read Buffer)/Channel 4/CH 4 // Verify Result Reg 0 - NTCNR_0X07E (V5A, V5CAN, 3V3, BUCK)/SetNtcSts/ISO Fault Debounce Design ==
  note: NTCSTS_PASSD           (0)
      | NTCSTS_FAILD             (1)
      | NTCSTS_PREPASSD   (2)
      | NTCSTS_PREFAILD     (3)
      |
      | SIGQLFR_NORES        (0)
      | SIGQLFR_PASSD         (1)
      | SIGQLFR_FAILD           (2)
  note: Pass Loop
  note: Fail Loop
  note: 
  (default) -> (junction 89)
  (junction 89) -> (junction 95) [order 1] : [NtcSts ==3]
  (junction 89) -> (junction 93) [order 2] : [NtcSts ==2]
  (junction 89) -> (junction 141) [order 3] : [NtcSts ==1]
      | { ErrAcc = 32767;
      | Qualifier =2;
      |  }
  (junction 89) -> (junction 141) [order 4] : [NtcSts ==0]
      | { ErrAcc = -32768;
      | Qualifier=1;
      | }
  (junction 95) -> (junction 103) [order 2]
  (junction 95) -> (junction 111) [order 1] : [ErrAcc <=0]
      | {ErrAcc = DebStep;}
  (junction 93) -> (junction 123) [order 2] : {
      | ErrAcc = ErrAcc - DebStep;
      | }
  (junction 93) -> (junction 123) [order 1] : [(ErrAcc - DebStep) <= -32768]
      | { ErrAcc = -32768;
      | Qualifier=1;
      | }
  (junction 103) -> (junction 111) [order 1] : [(ErrAcc + DebStep) <32767]
      | {ErrAcc = ErrAcc + DebStep;}
  (junction 103) -> (junction 111) [order 2] : {ErrAcc = 32767;
      | Qualifier =2;}
  (junction 123) -> (junction 141)
  (junction 111) -> (junction 141)
  (junction 141) -> (junction 159) [order 2] : {ErrAcc = 0;
      | Qualifier =0;
      | }
  (junction 141) -> (junction 159) [order 1] : [SvcClr ==0]
  data: NtcSts input uint8; Qualifier output uint8; DebStep input uint16; ErrAcc local int16; SvcClr input

== stateflow chart ES008A_PwrSply/PwrSply/PwrSplyPer1/SysSt = Enable/PwrSplyReadWrOrderFlg1 = 1 (Read Buffer)/CH 3 // Diag Reg 1 Error - NTCNR_0X07B (VREG, BUCK, V3V3)/SetNtcSts/ISO Fault Debounce Design ==
  note: NTCSTS_PASSD           (0)
      | NTCSTS_FAILD             (1)
      | NTCSTS_PREPASSD   (2)
      | NTCSTS_PREFAILD     (3)
      |
      | SIGQLFR_NORES        (0)
      | SIGQLFR_PASSD         (1)
      | SIGQLFR_FAILD           (2)
  note: Pass Loop
  note: Fail Loop
  note: 
  (default) -> (junction 89)
  (junction 89) -> (junction 95) [order 1] : [NtcSts ==3]
  (junction 89) -> (junction 93) [order 2] : [NtcSts ==2]
  (junction 89) -> (junction 141) [order 3] : [NtcSts ==1]
      | { ErrAcc = 32767;
      | Qualifier =2;
      |  }
  (junction 89) -> (junction 141) [order 4] : [NtcSts ==0]
      | { ErrAcc = -32768;
      | Qualifier=1;
      | }
  (junction 95) -> (junction 103) [order 2]
  (junction 95) -> (junction 111) [order 1] : [ErrAcc <=0]
      | {ErrAcc = DebStep;}
  (junction 93) -> (junction 123) [order 2] : {
      | ErrAcc = ErrAcc - DebStep;
      | }
  (junction 93) -> (junction 123) [order 1] : [(ErrAcc - DebStep) <= -32768]
      | { ErrAcc = -32768;
      | Qualifier=1;
      | }
  (junction 103) -> (junction 111) [order 1] : [(ErrAcc + DebStep) <32767]
      | {ErrAcc = ErrAcc + DebStep;}
  (junction 103) -> (junction 111) [order 2] : {ErrAcc = 32767;
      | Qualifier =2;}
  (junction 123) -> (junction 141)
  (junction 111) -> (junction 141)
  (junction 141) -> (junction 159) [order 2] : {ErrAcc = 0;
      | Qualifier =0;
      | }
  (junction 141) -> (junction 159) [order 1] : [SvcClr ==0]
  data: NtcSts input uint8; Qualifier output uint8; DebStep input uint16; ErrAcc local int16; SvcClr input

== stateflow chart ES008A_PwrSply/PwrSply/PwrSplyPer1/SysSt = Enable/PwrSplyReadWrOrderFlg1 = 1 (Read Buffer)/No  Error - Diag Reg 1/SetNtcSts/ISO Fault Debounce Design ==
  note: NTCSTS_PASSD           (0)
      | NTCSTS_FAILD             (1)
      | NTCSTS_PREPASSD   (2)
      | NTCSTS_PREFAILD     (3)
      |
      | SIGQLFR_NORES        (0)
      | SIGQLFR_PASSD         (1)
      | SIGQLFR_FAILD           (2)
  note: Pass Loop
  note: Fail Loop
  note: 
  (default) -> (junction 89)
  (junction 89) -> (junction 95) [order 1] : [NtcSts ==3]
  (junction 89) -> (junction 93) [order 2] : [NtcSts ==2]
  (junction 89) -> (junction 141) [order 3] : [NtcSts ==1]
      | { ErrAcc = 32767;
      | Qualifier =2;
      |  }
  (junction 89) -> (junction 141) [order 4] : [NtcSts ==0]
      | { ErrAcc = -32768;
      | Qualifier=1;
      | }
  (junction 95) -> (junction 103) [order 2]
  (junction 95) -> (junction 111) [order 1] : [ErrAcc <=0]
      | {ErrAcc = DebStep;}
  (junction 93) -> (junction 123) [order 2] : {
      | ErrAcc = ErrAcc - DebStep;
      | }
  (junction 93) -> (junction 123) [order 1] : [(ErrAcc - DebStep) <= -32768]
      | { ErrAcc = -32768;
      | Qualifier=1;
      | }
  (junction 103) -> (junction 111) [order 1] : [(ErrAcc + DebStep) <32767]
      | {ErrAcc = ErrAcc + DebStep;}
  (junction 103) -> (junction 111) [order 2] : {ErrAcc = 32767;
      | Qualifier =2;}
  (junction 123) -> (junction 141)
  (junction 111) -> (junction 141)
  (junction 141) -> (junction 159) [order 2] : {ErrAcc = 0;
      | Qualifier =0;
      | }
  (junction 141) -> (junction 159) [order 1] : [SvcClr ==0]
  data: NtcSts input uint8; Qualifier output uint8; DebStep input uint16; ErrAcc local int16; SvcClr input

== stateflow chart ES008A_PwrSply/PwrSply/PwrSplyPer1/SysSt = Enable/PwrSplyReadWrOrderFlg1 = 1 (Read Buffer)/CH 2 // Diag Reg 0 Error - NTCNR_0X07C (V5P, V5A, V5B, V5CAN)/SetNtcSts/ISO Fault Debounce Design ==
  note: NTCSTS_PASSD           (0)
      | NTCSTS_FAILD             (1)
      | NTCSTS_PREPASSD   (2)
      | NTCSTS_PREFAILD     (3)
      |
      | SIGQLFR_NORES        (0)
      | SIGQLFR_PASSD         (1)
      | SIGQLFR_FAILD           (2)
  note: Pass Loop
  note: Fail Loop
  note: 
  (default) -> (junction 89)
  (junction 89) -> (junction 95) [order 1] : [NtcSts ==3]
  (junction 89) -> (junction 93) [order 2] : [NtcSts ==2]
  (junction 89) -> (junction 141) [order 3] : [NtcSts ==1]
      | { ErrAcc = 32767;
      | Qualifier =2;
      |  }
  (junction 89) -> (junction 141) [order 4] : [NtcSts ==0]
      | { ErrAcc = -32768;
      | Qualifier=1;
      | }
  (junction 95) -> (junction 103) [order 2]
  (junction 95) -> (junction 111) [order 1] : [ErrAcc <=0]
      | {ErrAcc = DebStep;}
  (junction 93) -> (junction 123) [order 2] : {
      | ErrAcc = ErrAcc - DebStep;
      | }
  (junction 93) -> (junction 123) [order 1] : [(ErrAcc - DebStep) <= -32768]
      | { ErrAcc = -32768;
      | Qualifier=1;
      | }
  (junction 103) -> (junction 111) [order 1] : [(ErrAcc + DebStep) <32767]
      | {ErrAcc = ErrAcc + DebStep;}
  (junction 103) -> (junction 111) [order 2] : {ErrAcc = 32767;
      | Qualifier =2;}
  (junction 123) -> (junction 141)
  (junction 111) -> (junction 141)
  (junction 141) -> (junction 159) [order 2] : {ErrAcc = 0;
      | Qualifier =0;
      | }
  (junction 141) -> (junction 159) [order 1] : [SvcClr ==0]
  data: NtcSts input uint8; Qualifier output uint8; DebStep input uint16; ErrAcc local int16; SvcClr input

== stateflow chart ES008A_PwrSply/PwrSply/PwrSplyPer1/SysSt = Warm Init OR Enable/PwrSplyReadWrOrderFlg2 = 1 (Read Buffer)/Channel 5/CH 5 // Verify Result Reg 1 - NTCNR_0X07F (VREG, V5P, V5B)/SetNtcSts/ISO Fault Debounce Design ==
  note: NTCSTS_PASSD           (0)
      | NTCSTS_FAILD             (1)
      | NTCSTS_PREPASSD   (2)
      | NTCSTS_PREFAILD     (3)
      |
      | SIGQLFR_NORES        (0)
      | SIGQLFR_PASSD         (1)
      | SIGQLFR_FAILD           (2)
  note: Pass Loop
  note: Fail Loop
  note: 
  (default) -> (junction 89)
  (junction 89) -> (junction 95) [order 1] : [NtcSts ==3]
  (junction 89) -> (junction 93) [order 2] : [NtcSts ==2]
  (junction 89) -> (junction 141) [order 3] : [NtcSts ==1]
      | { ErrAcc = 32767;
      | Qualifier =2;
      |  }
  (junction 89) -> (junction 141) [order 4] : [NtcSts ==0]
      | { ErrAcc = -32768;
      | Qualifier=1;
      | }
  (junction 95) -> (junction 103) [order 2]
  (junction 95) -> (junction 111) [order 1] : [ErrAcc <=0]
      | {ErrAcc = DebStep;}
  (junction 93) -> (junction 123) [order 2] : {
      | ErrAcc = ErrAcc - DebStep;
      | }
  (junction 93) -> (junction 123) [order 1] : [(ErrAcc - DebStep) <= -32768]
      | { ErrAcc = -32768;
      | Qualifier=1;
      | }
  (junction 103) -> (junction 111) [order 1] : [(ErrAcc + DebStep) <32767]
      | {ErrAcc = ErrAcc + DebStep;}
  (junction 103) -> (junction 111) [order 2] : {ErrAcc = 32767;
      | Qualifier =2;}
  (junction 123) -> (junction 141)
  (junction 111) -> (junction 141)
  (junction 141) -> (junction 159) [order 2] : {ErrAcc = 0;
      | Qualifier =0;
      | }
  (junction 141) -> (junction 159) [order 1] : [SvcClr ==0]
  data: NtcSts input uint8; Qualifier output uint8; DebStep input uint16; ErrAcc local int16; SvcClr input

== stateflow chart ES008A_PwrSply/PwrSply/PwrSplyPer1/SysSt = Warm Init OR Enable/PwrSplyReadWrOrderFlg2 = 1 (Read Buffer)/Channel 5/No Startup Test Error 1/SetNtcSts/ISO Fault Debounce Design ==
  note: NTCSTS_PASSD           (0)
      | NTCSTS_FAILD             (1)
      | NTCSTS_PREPASSD   (2)
      | NTCSTS_PREFAILD     (3)
      |
      | SIGQLFR_NORES        (0)
      | SIGQLFR_PASSD         (1)
      | SIGQLFR_FAILD           (2)
  note: Pass Loop
  note: Fail Loop
  note: 
  (default) -> (junction 89)
  (junction 89) -> (junction 95) [order 1] : [NtcSts ==3]
  (junction 89) -> (junction 93) [order 2] : [NtcSts ==2]
  (junction 89) -> (junction 141) [order 3] : [NtcSts ==1]
      | { ErrAcc = 32767;
      | Qualifier =2;
      |  }
  (junction 89) -> (junction 141) [order 4] : [NtcSts ==0]
      | { ErrAcc = -32768;
      | Qualifier=1;
      | }
  (junction 95) -> (junction 103) [order 2]
  (junction 95) -> (junction 111) [order 1] : [ErrAcc <=0]
      | {ErrAcc = DebStep;}
  (junction 93) -> (junction 123) [order 2] : {
      | ErrAcc = ErrAcc - DebStep;
      | }
  (junction 93) -> (junction 123) [order 1] : [(ErrAcc - DebStep) <= -32768]
      | { ErrAcc = -32768;
      | Qualifier=1;
      | }
  (junction 103) -> (junction 111) [order 1] : [(ErrAcc + DebStep) <32767]
      | {ErrAcc = ErrAcc + DebStep;}
  (junction 103) -> (junction 111) [order 2] : {ErrAcc = 32767;
      | Qualifier =2;}
  (junction 123) -> (junction 141)
  (junction 111) -> (junction 141)
  (junction 141) -> (junction 159) [order 2] : {ErrAcc = 0;
      | Qualifier =0;
      | }
  (junction 141) -> (junction 159) [order 1] : [SvcClr ==0]
  data: NtcSts input uint8; Qualifier output uint8; DebStep input uint16; ErrAcc local int16; SvcClr input

== stateflow chart ES008A_PwrSply/PwrSply/PwrSplyPer1/SysSt = Enable/PwrSplyReadWrOrderFlg1 = 1 (Read Buffer)/No  Error - Diag Reg 0/SetNtcSts/ISO Fault Debounce Design ==
  note: NTCSTS_PASSD           (0)
      | NTCSTS_FAILD             (1)
      | NTCSTS_PREPASSD   (2)
      | NTCSTS_PREFAILD     (3)
      |
      | SIGQLFR_NORES        (0)
      | SIGQLFR_PASSD         (1)
      | SIGQLFR_FAILD           (2)
  note: Pass Loop
  note: Fail Loop
  note: 
  (default) -> (junction 89)
  (junction 89) -> (junction 95) [order 1] : [NtcSts ==3]
  (junction 89) -> (junction 93) [order 2] : [NtcSts ==2]
  (junction 89) -> (junction 141) [order 3] : [NtcSts ==1]
      | { ErrAcc = 32767;
      | Qualifier =2;
      |  }
  (junction 89) -> (junction 141) [order 4] : [NtcSts ==0]
      | { ErrAcc = -32768;
      | Qualifier=1;
      | }
  (junction 95) -> (junction 103) [order 2]
  (junction 95) -> (junction 111) [order 1] : [ErrAcc <=0]
      | {ErrAcc = DebStep;}
  (junction 93) -> (junction 123) [order 2] : {
      | ErrAcc = ErrAcc - DebStep;
      | }
  (junction 93) -> (junction 123) [order 1] : [(ErrAcc - DebStep) <= -32768]
      | { ErrAcc = -32768;
      | Qualifier=1;
      | }
  (junction 103) -> (junction 111) [order 1] : [(ErrAcc + DebStep) <32767]
      | {ErrAcc = ErrAcc + DebStep;}
  (junction 103) -> (junction 111) [order 2] : {ErrAcc = 32767;
      | Qualifier =2;}
  (junction 123) -> (junction 141)
  (junction 111) -> (junction 141)
  (junction 141) -> (junction 159) [order 2] : {ErrAcc = 0;
      | Qualifier =0;
      | }
  (junction 141) -> (junction 159) [order 1] : [SvcClr ==0]
  data: NtcSts input uint8; Qualifier output uint8; DebStep input uint16; ErrAcc local int16; SvcClr input

== stateflow chart ES008A_PwrSply/PwrSply/PwrSplyPer1/SysSt = Enable/PwrSplyReadWrOrderFlg1 = 1 (Read Buffer)/Serial Error - NTCNR_0X07D/SetNtcSts/ISO Fault Debounce Design ==
  note: NTCSTS_PASSD           (0)
      | NTCSTS_FAILD             (1)
      | NTCSTS_PREPASSD   (2)
      | NTCSTS_PREFAILD     (3)
      |
      | SIGQLFR_NORES        (0)
      | SIGQLFR_PASSD         (1)
      | SIGQLFR_FAILD           (2)
  note: Pass Loop
  note: Fail Loop
  note: 
  (default) -> (junction 89)
  (junction 89) -> (junction 95) [order 1] : [NtcSts ==3]
  (junction 89) -> (junction 93) [order 2] : [NtcSts ==2]
  (junction 89) -> (junction 141) [order 3] : [NtcSts ==1]
      | { ErrAcc = 32767;
      | Qualifier =2;
      |  }
  (junction 89) -> (junction 141) [order 4] : [NtcSts ==0]
      | { ErrAcc = -32768;
      | Qualifier=1;
      | }
  (junction 95) -> (junction 103) [order 2]
  (junction 95) -> (junction 111) [order 1] : [ErrAcc <=0]
      | {ErrAcc = DebStep;}
  (junction 93) -> (junction 123) [order 2] : {
      | ErrAcc = ErrAcc - DebStep;
      | }
  (junction 93) -> (junction 123) [order 1] : [(ErrAcc - DebStep) <= -32768]
      | { ErrAcc = -32768;
      | Qualifier=1;
      | }
  (junction 103) -> (junction 111) [order 1] : [(ErrAcc + DebStep) <32767]
      | {ErrAcc = ErrAcc + DebStep;}
  (junction 103) -> (junction 111) [order 2] : {ErrAcc = 32767;
      | Qualifier =2;}
  (junction 123) -> (junction 141)
  (junction 111) -> (junction 141)
  (junction 141) -> (junction 159) [order 2] : {ErrAcc = 0;
      | Qualifier =0;
      | }
  (junction 141) -> (junction 159) [order 1] : [SvcClr ==0]
  data: NtcSts input uint8; Qualifier output uint8; DebStep input uint16; ErrAcc local int16; SvcClr input

== stateflow chart ES008A_PwrSply/PwrSply/PwrSplyPer1/SysSt = Enable/PwrSplyReadWrOrderFlg1 = 1 (Read Buffer)/No Serial Error/SetNtcSts/ISO Fault Debounce Design ==
  note: NTCSTS_PASSD           (0)
      | NTCSTS_FAILD             (1)
      | NTCSTS_PREPASSD   (2)
      | NTCSTS_PREFAILD     (3)
      |
      | SIGQLFR_NORES        (0)
      | SIGQLFR_PASSD         (1)
      | SIGQLFR_FAILD           (2)
  note: Pass Loop
  note: Fail Loop
  note: 
  (default) -> (junction 89)
  (junction 89) -> (junction 95) [order 1] : [NtcSts ==3]
  (junction 89) -> (junction 93) [order 2] : [NtcSts ==2]
  (junction 89) -> (junction 141) [order 3] : [NtcSts ==1]
      | { ErrAcc = 32767;
      | Qualifier =2;
      |  }
  (junction 89) -> (junction 141) [order 4] : [NtcSts ==0]
      | { ErrAcc = -32768;
      | Qualifier=1;
      | }
  (junction 95) -> (junction 103) [order 2]
  (junction 95) -> (junction 111) [order 1] : [ErrAcc <=0]
      | {ErrAcc = DebStep;}
  (junction 93) -> (junction 123) [order 2] : {
      | ErrAcc = ErrAcc - DebStep;
      | }
  (junction 93) -> (junction 123) [order 1] : [(ErrAcc - DebStep) <= -32768]
      | { ErrAcc = -32768;
      | Qualifier=1;
      | }
  (junction 103) -> (junction 111) [order 1] : [(ErrAcc + DebStep) <32767]
      | {ErrAcc = ErrAcc + DebStep;}
  (junction 103) -> (junction 111) [order 2] : {ErrAcc = 32767;
      | Qualifier =2;}
  (junction 123) -> (junction 141)
  (junction 111) -> (junction 141)
  (junction 141) -> (junction 159) [order 2] : {ErrAcc = 0;
      | Qualifier =0;
      | }
  (junction 141) -> (junction 159) [order 1] : [SvcClr ==0]
  data: NtcSts input uint8; Qualifier output uint8; DebStep input uint16; ErrAcc local int16; SvcClr input
